simulink model "waiper"  (R2015b)
settings: Solver=FixedStepDiscrete  StartTime=0.0  StopTime=10  FixedStep=0.01  RelTol=1e-3
undefined symbols (not defined in the file): sigbuilder_block
settings Model: Creator=studypc2  LastModifiedBy=admin-cs
settings DataIOCC: SaveFormat=Array  SignalLogging=off
settings OptimizationCC: ExpressionDepthLimit=2147483647
settings DebuggingCC: UnderspecifiedInitializationDetection=Classic  MergeDetectMultiDrivingBlocksExec=none  SolverPrmCheckMsg=warning  StateNameClashWarn=warning
settings HardwareCC: ProdBitPerPointer=32  ProdLargestAtomicFloat=None  ProdIntDivRoundTo=Undefined  ProdEndianess=Unspecified  ProdWordSize=32  ProdHWDeviceType=32-bit Generic
settings GRTTargetCC: GeneratePreprocessorConditionals=Disable all
settings ConfigComp: CovModelRefEnable=Off

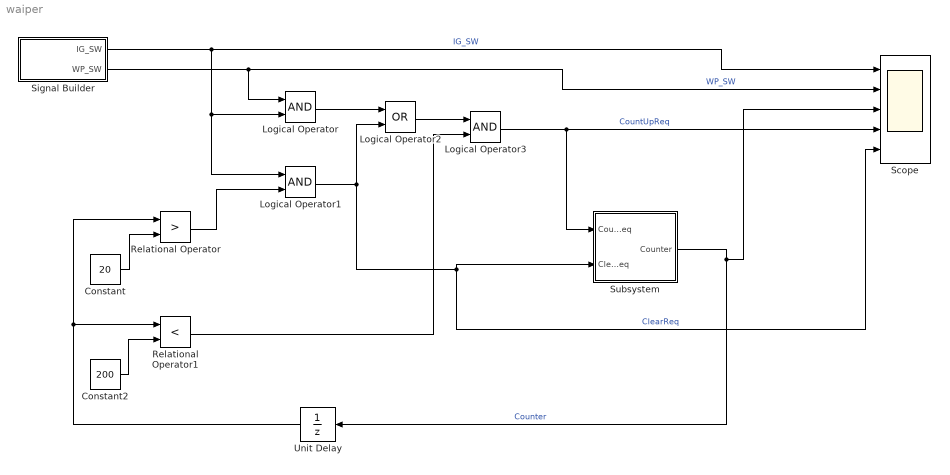
== system waiper ==
  Constant : Constant  Value=20
  Constant2 : Constant  Value=200
  Logical Operator : Logic  AllPortsSameDT=off  OutDataTypeStr=boolean
  Logical Operator1 : Logic  AllPortsSameDT=off  OutDataTypeStr=boolean
  Logical Operator2 : Logic  Operator=OR  AllPortsSameDT=off  OutDataTypeStr=boolean
  Logical Operator3 : Logic  AllPortsSameDT=off  OutDataTypeStr=boolean
  Relational Operator : RelationalOperator  Operator=>  OutDataTypeStr=boolean
  Relational Operator1 : RelationalOperator  Operator=<  OutDataTypeStr=boolean
  Scope : Scope  NumInputPorts=5
  Signal Builder : Subsystem  Tag=STV Subsys  LoadFcn=sigbuilder_block('load');  StartFcn=sigbuilder_block('start');  StopFcn=sigbuilder_block('stop');  ClipboardFcn=sigbuilder_block('clipboard');  mask(Sigbuilder block){}
      mask help: Simulink:masks:SigbuilderBlock_MD
      mask init:
      | if ~strcmp(get_param(bdroot(gcbh),'SimulationStatus'),'stopped') tuvar = sigbuilder_block('maskInit'); end
      settings: CopyFcn=sigbuilder_block('copy');  DeleteFcn=sigbuilder_block('delete');  ModelCloseFcn=sigbuilder_block('modelClose');  PreSaveFcn=sigbuilder_block('preSave');  PauseFcn=sigbuilder_block('pause');  ContinueFcn=sigbuilder_block('continue');  NameChangeFcn=sigbuilder_block('namechange');  OpenFcn=sigbuilder_block('open',[249.75 69 738 441.75 ]);  CloseFcn=sigbuilder_block('close');
      mask Display: plot(0, 0, 100, 100,[2, 2, 32, 32, 2], [68, 8, 8, 68, 68],[32, 2], [38, 38], [32, 19, 2],[53, 60, 44], [32, 17, 17, 2],[16, 16, 31, 31]);txt = getActiveGroup(gcbh);text(2, 100, txt,'verticalAlignment', 'top');
  Subsystem : Subsystem
  Unit Delay : UnitDelay  SampleTime=-1
  wires:
  Logical Operator3/1 -> Subsystem/1(CountUpReq), Scope/4  "CountUpReq"
  Subsystem/1(Counter) -> Unit Delay/1, Scope/3  "Counter"
  Logical Operator1/1 -> Logical Operator2/2, Scope/5, Subsystem/2(ClearReq)  "ClearReq"
  Signal Builder/1(IG_SW) -> Logical Operator1/1, Logical Operator/2, Scope/1  "IG_SW"
  Signal Builder/2(WP_SW) -> Scope/2, Logical Operator/1  "WP_SW"
  Logical Operator/1 -> Logical Operator2/1
  Logical Operator2/1 -> Logical Operator3/1
  Relational Operator/1 -> Logical Operator1/2
  Constant/1 -> Relational Operator/2
  Constant2/1 -> Relational Operator1/2
  Unit Delay/1 -> Relational Operator1/1, Relational Operator/1
  Relational Operator1/1 -> Logical Operator3/2

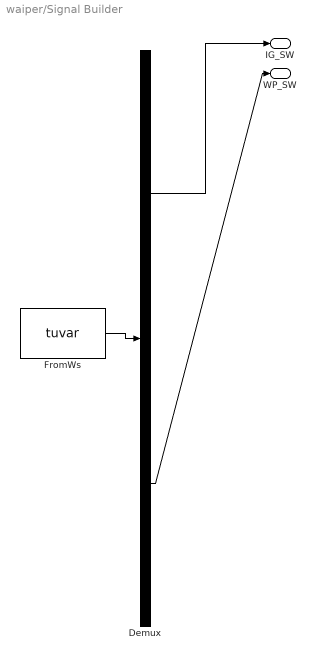
== system waiper/Signal Builder ==
  Demux : Demux  Tag=STV Demux  Outputs=2
  FromWs : FromWorkspace  Tag=STV FromWs  VariableName=tuvar  SampleTime=0
      SigBuilderData=|
      | common.afterFinalStr = 'Extrapolate'
      | common.sampleTime = 0
      | dataSet.timeRange = [0 10]
      | dataSet.name = 'Group 1'
      | sbobj.Groups.Name = 'Group 1'
      | sbobj.Groups.Signals(1).Name = 'IG_SW'
      | sbobj.Groups.Signals(1).XData = [0 0.54 0.54 4.98 6.84 6.84 7.58 7.58 9.46 9.46 10]
      | sbobj.Groups.Signals(1).YData = [-0.01 -0.01 0.99 0.99 0.99 -0.01 -0.01 0.99 0.99 -0.01 -0.01]
      | sbobj.Groups.Signals(2).Name = 'WP_SW'
      | sbobj.Groups.Signals(2).XData = [0 0.92 0.92 3.26 3.26 5.52 5.52 5.66 5.66 6.36 6.36 9.04 9.04 10]
      | sbobj.Groups.Signals(2).YData = [0 0 1 1 0 0 1 1 0 0 1 1 0 0]
  IG_SW : Outport  Tag=STV Outport
  WP_SW : Outport  Tag=STV Outport  Port=2
  wires:
  Demux/1 -> IG_SW/1
  FromWs/1 -> Demux/1
  Demux/2 -> WP_SW/1

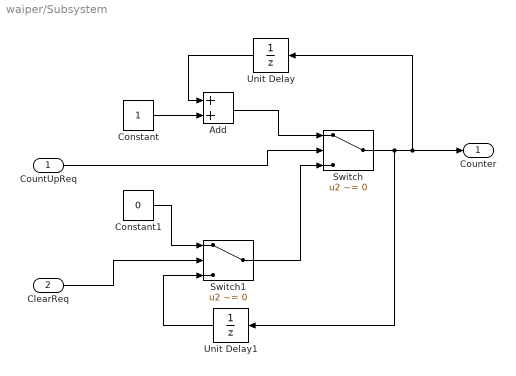
== system waiper/Subsystem ==
  CountUpReq : Inport
  ClearReq : Inport  Port=2
  Add : Sum
  Constant : Constant  OutDataTypeStr=double
  Constant1 : Constant  Value=0  OutDataTypeStr=double
  Switch : Switch  Criteria=u2 ~= 0
  Switch1 : Switch  Criteria=u2 ~= 0
  Unit Delay : UnitDelay  SampleTime=-1
  Unit Delay1 : UnitDelay  SampleTime=-1
  Counter : Outport
  wires:
  Switch1/1 -> Switch/3
  Constant/1 -> Add/2
  Add/1 -> Switch/1
  CountUpReq/1 -> Switch/2
  Constant1/1 -> Switch1/1
  Switch/1 -> Unit Delay1/1, Counter/1, Unit Delay/1
  Unit Delay/1 -> Add/1
  Unit Delay1/1 -> Switch1/3
  ClearReq/1 -> Switch1/2
